simulink model "Winkelregelung44bb"  (R2017a)
settings: Solver=VariableStepAuto  StartTime=0.0  StopTime=10.0  RelTol=1e-3
undefined symbols (not defined in the file): g, kfy, kvy, mc, mw, R, Ra, Ry
settings Model: Creator=prt01  LastModifiedBy=prt01

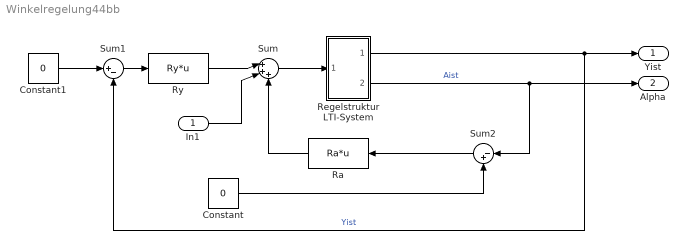
== system Winkelregelung44bb ==
  In1 : Inport
  Constant : Constant  Value=0
  Constant1 : Constant  Value=0
  Ra : Fcn  Expr=Ra*u
  Regelstruktur LTI-System : Subsystem
  Ry : Fcn  Expr=Ry*u
  Sum : Sum  Inputs=|+++
  Sum1 : Sum  Inputs=|+-
  Sum2 : Sum  Inputs=|-+
  Yist : Outport
  Alpha : Outport  Port=2
  wires:
  Regelstruktur LTI-System/1(Out1) -> Sum1/2, Yist/1  "Yist"
  Regelstruktur LTI-System/2(Out2) -> Sum2/1, Alpha/1  "Aist"
  Sum/1 -> Regelstruktur LTI-System/1(In1)
  Constant1/1 -> Sum1/1
  Sum1/1 -> Ry/1
  Ry/1 -> Sum/1
  Sum2/1 -> Ra/1
  Constant/1 -> Sum2/2
  Ra/1 -> Sum/3
  In1/1 -> Sum/2

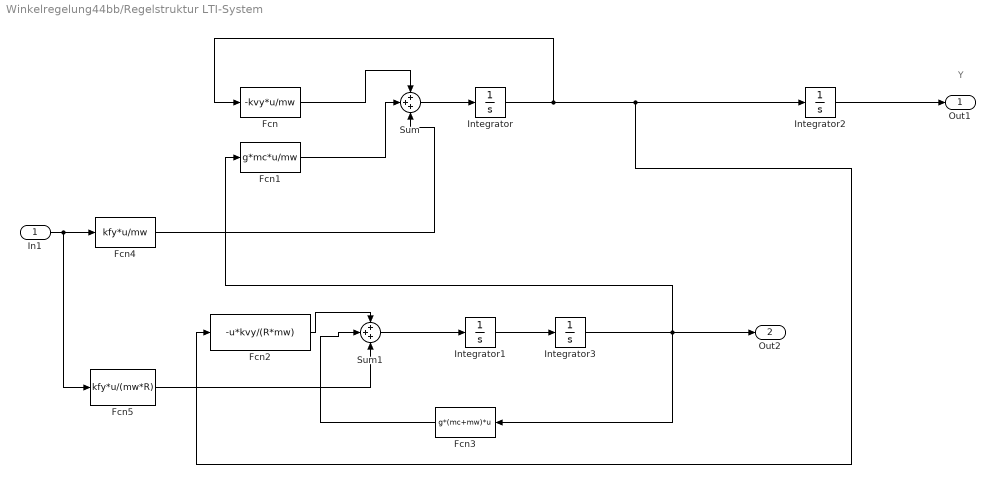
== system Winkelregelung44bb/Regelstruktur LTI-System ==
  note: Y
  In1 : Inport
  Fcn : Fcn  Expr=-kvy*u/mw
  Fcn1 : Fcn  Expr=g*mc*u/mw
  Fcn2 : Fcn  Expr=-u*kvy/(R*mw)
  Fcn3 : Fcn  Expr=g*(mc+mw)*u
  Fcn4 : Fcn  Expr=kfy*u/mw
  Fcn5 : Fcn  Expr=kfy*u/(mw*R)
  Integrator{,1..3} (4 alike) : Integrator
  Sum : Sum  Inputs=+++
  Sum1 : Sum  Inputs=+++
  Out1 : Outport
  Out2 : Outport  Port=2
  wires:
  Fcn1/1 -> Sum/2
  Integrator/1 -> Fcn/1, Fcn2/1, Integrator2/1
  Fcn2/1 -> Sum1/1
  Sum/1 -> Integrator/1
  Integrator1/1 -> Integrator3/1
  Integrator3/1 -> Fcn3/1, Out2/1, Fcn1/1
  Integrator2/1 -> Out1/1
  Fcn3/1 -> Sum1/2
  Sum1/1 -> Integrator1/1
  Fcn/1 -> Sum/1
  In1/1 -> Fcn5/1, Fcn4/1
  Fcn4/1 -> Sum/3
  Fcn5/1 -> Sum1/3
